simulink library "ANTlib"  (Simulink 5.0)
libraries: simulink x3
settings Model: LastModifiedBy=Тукмачев А Н

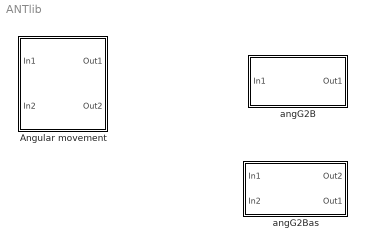
== system ANTlib ==
  Angular movement : Subsystem  mask(Angular movement){}
      mask help:
      | Vector VJ=[Jxx, Jyy, Jzz, Jxy, Jyz, Jxz];
      | Ang_g=[fie psi tet];
      mask init:
      | g=(1:40)*pi/30;
      | y=sin(g)/5+0.5;
      | x=cos(g)/5+0.5;
      mask Display:
      | port_label('input',1,'M');
      | port_label('input',2,'VJ');
      | port_label('output',1,'Omega');
      | port_label('output',2,'Ang_g');
      | plot(x,y);
      | patch([.64 .75 .69 .64],[.5 .5 .4 .5]);
  angG2B : Subsystem
      mask Type: angG2B
      mask Description: [fie psi tet]>>>B
      mask Display:
      | port_label('input',1,'Ang_fpt')
      | port_label('output',1,'B')
      | disp('          A_g2B')
  angG2Bas : Subsystem
      mask Type: angG2Bas
      mask Description: Расчет матрицы B по углам и с-углов
      mask Display:
      | port_label('input',1,'Ang_fpt')
      | port_label('output',2,'B')
      | port_label('output',1,'AngS')
      | disp('Ang2Bas')
      | port_label('input',2,'Bpr')

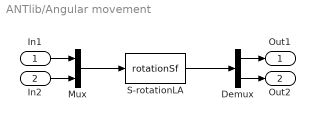
== system ANTlib/Angular movement ==
  In1 : Inport
  In2 : Inport  Port=2
  Demux : Demux  Outputs=2
  Mux : Mux  Inputs=2
  S-rotationLA : S-Function  FunctionName=rotationSf  Parameters=AnStart
  Out1 : Outport
  Out2 : Outport  Port=2
  wires:
  Mux/1 -> S-rotationLA/1
  S-rotationLA/1 -> Demux/1
  Demux/1 -> Out1/1
  In1/1 -> Mux/1
  Demux/2 -> Out2/1
  In2/1 -> Mux/2

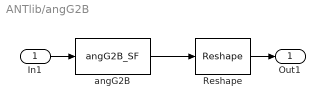
== system ANTlib/angG2B ==
  In1 : Inport
  Reshape : simulink/Math Operations/Reshape  OutputDimensionality=Customize  OutputDimensions=[3,3]
  angG2B : S-Function  FunctionName=angG2B_SF
  Out1 : Outport
  wires:
  angG2B/1 -> Reshape/1
  Reshape/1 -> Out1/1
  In1/1 -> angG2B/1

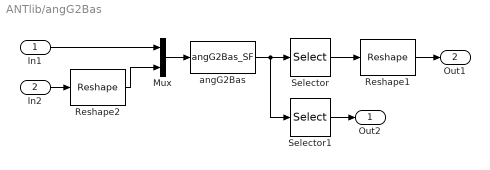
== system ANTlib/angG2Bas ==
  In1 : Inport
  In2 : Inport  Port=2
  Mux : Mux  Inputs=2
  Reshape1 : simulink/Math Operations/Reshape  OutputDimensionality=Customize  OutputDimensions=[3,3]
  Reshape2 : simulink/Math Operations/Reshape  OutputDimensionality=Column vector  OutputDimensions=[3,3]
  Selector : Selector  Elements=[1:9]  InputPortWidth=12
  Selector1 : Selector  Elements=[10 :12]  InputPortWidth=12
  angG2Bas : S-Function  FunctionName=angG2Bas_SF
  Out2 : Outport
  Out1 : Outport  Port=2
  wires:
  angG2Bas/1 -> Selector/1, Selector1/1
  Selector/1 -> Reshape1/1
  Reshape1/1 -> Out1/1
  Selector1/1 -> Out2/1
  In2/1 -> Reshape2/1
  Mux/1 -> angG2Bas/1
  In1/1 -> Mux/1
  Reshape2/1 -> Mux/2
